simulink model "OpticflowRotation_mod"  (Simulink 7.6)
settings: Solver=ode45  StartTime=0.0  StopTime=inf  FixedStep=1  RelTol=1e-3
undefined symbols (not defined in the file or in its folder): Horn, jet, none, Schunck, videoinput
libraries: dspstat3 x6, simulink x3, dspmtrx3 x2, vipanalysis x2, imaqlib x1, vipsnks x1
settings Model: Creator=pacifist  LastModifiedBy=Administrator
settings SimEventsCC: propDiagAttribOutput=1  propDiagFcnCallOutput=1  propDiagStatOutput=0

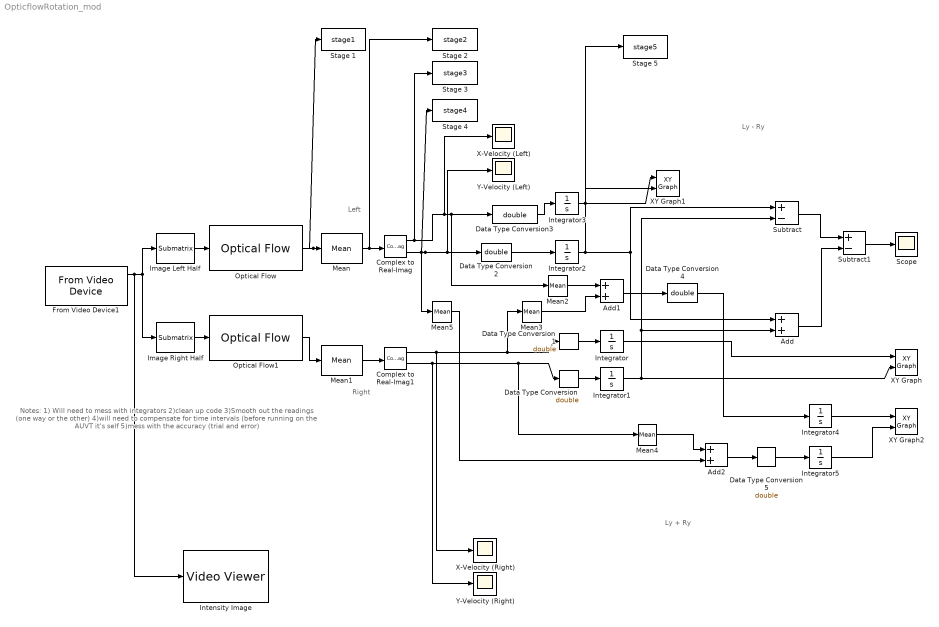
== system OpticflowRotation_mod ==
  note: Notes:
      | 1) Will need to mess with integrators
      | 2)clean up code
      | 3)Smooth out the readings (one way or the other)
      | 4)will need to compensate for time intervals (before running on the AUVT it's self
      | 5)mess with the accuracy (trial and error)
  note: Right
  note: Left
  note: Ly - Ry
  note: Ly + Ry
  Add : Sum
  Add1 : Sum
  Add2 : Sum
  Complex to Real-Imag : ComplexToRealImag
  Complex to Real-Imag1 : ComplexToRealImag
  Data Type Conversion{,1..5} (6 alike) : DataTypeConversion  OutDataTypeStr=double
  From Video Device1 : imaqlib/From Video Device  DialogController=imaqcreatedialog  DialogControllerArgs=DataTag1  DeviceMenu=winvideo 1 (VC0334 USB2.0 Digital Camera)  Device=winvideo 1 (VC0334 USB2.0 Digital Camera)  ObjConstructor=videoinput('winvideo', 1)  VideoFormatMenu=I420_160x120  VideoFormat=I420_160x120  VideoSource=input1  ROIPosition=[0 0 120 160]  EnableHWTrigger=off  TriggerConfiguration=none/none  SampleTime=1/30  OutputPortsMode=Separate color signals  DataType=single  CanDoHWTrigger=no  ReturnedColorSpace=YCbCr  BlockHandle=1940.0005  ROIWidth=160  ROIHeight=120  ROIColumn=0  ROIRow=0  EngXMLPath=C:\Program Files\MATLAB\R2010b\toolbox\imaq\imaq\private  DevXMLPath=C:\Program Files\MATLAB\R2010b\toolbox\imaq\imaqadaptors\win32  EngLibPath=C:\Program Files\MATLAB\R2010b\toolbox\imaq\imaqblks\imaqmex\win32
  Image Left Half : dspmtrx3/Submatrix  RowSpan=All rows  RowStartMode=First  RowStartIndex=1  RowEndMode=Last  RowEndIndex=1  ColSpan=Range of columns  ColStartMode=First  ColStartIndex=1  ColEndMode=Offset from middle  ColEndIndex=-1
  Image Right Half : dspmtrx3/Submatrix  RowSpan=All rows  RowStartMode=First  RowStartIndex=1  RowEndMode=Last  RowEndIndex=1  ColSpan=Range of columns  ColStartMode=Middle  ColStartIndex=1  ColEndMode=Last  ColEndIndex=1
  Integrator{,1..5} (6 alike) : Integrator  LimitOutput=on  UpperSaturationLimit=.01  LowerSaturationLimit=-.01
  Intensity Image : vipsnks/Video Viewer  DialogControllerArgs=DataTag3  inputType=Obsolete7b  imagePorts=One multidimensional signal  useColorMap=off  colormapValue=jet(256)  specRange=off  minInputVal=0  maxInputVal=255  FigPos=[691 710 267 180]  AxisZoom=on  trueSizedOnce=off  OpenAtMdlStart=on
  Mean : dspstat3/Mean  DialogController=dspDDGCreate  DialogControllerArgs=DataTag5  run=off  reset_popup=None  InputProcessing=Columns as channels (frame based)  directionMode=Entire input  dimension=1  treatSBRowAsCol=on  roiEnable=off  roiType=Rectangles  roiPortion=Entire ROI  roiOutput=Individual statistics for each ROI  roiFlag=off  outputDataTypeStr=Inherit: Same as accumulator  outputLastDataTypeStr=Inherit: Same as accumulator  outputMin=[]  outputMax=[]  roundingMode=Floor  overflowMode=off
  Mean1 : dspstat3/Mean  DialogController=dspDDGCreate  DialogControllerArgs=DataTag7  run=off  reset_popup=None  InputProcessing=Columns as channels (frame based)  directionMode=Entire input  dimension=1  treatSBRowAsCol=on  roiEnable=off  roiType=Rectangles  roiPortion=Entire ROI  roiOutput=Individual statistics for each ROI  roiFlag=off  outputDataTypeStr=Inherit: Same as accumulator  outputLastDataTypeStr=Inherit: Same as accumulator  outputMin=[]  outputMax=[]  roundingMode=Floor  overflowMode=off
  Mean2 : dspstat3/Mean  DialogController=dspDDGCreate  DialogControllerArgs=DataTag9  run=off  reset_popup=None  InputProcessing=Columns as channels (frame based)  directionMode=Entire input  dimension=1  treatSBRowAsCol=on  roiEnable=off  roiType=Rectangles  roiPortion=Entire ROI  roiOutput=Individual statistics for each ROI  roiFlag=off  outputDataTypeStr=Inherit: Same as accumulator  outputLastDataTypeStr=Inherit: Same as accumulator  outputMin=[]  outputMax=[]  roundingMode=Floor  overflowMode=off
  Mean3 : dspstat3/Mean  DialogController=dspDDGCreate  DialogControllerArgs=DataTag11  run=off  reset_popup=None  InputProcessing=Columns as channels (frame based)  directionMode=Entire input  dimension=1  treatSBRowAsCol=on  roiEnable=off  roiType=Rectangles  roiPortion=Entire ROI  roiOutput=Individual statistics for each ROI  roiFlag=off  outputDataTypeStr=Inherit: Same as accumulator  outputLastDataTypeStr=Inherit: Same as accumulator  outputMin=[]  outputMax=[]  roundingMode=Floor  overflowMode=off
  Mean4 : dspstat3/Mean  DialogController=dspDDGCreate  DialogControllerArgs=DataTag13  run=off  reset_popup=None  InputProcessing=Columns as channels (frame based)  directionMode=Entire input  dimension=1  treatSBRowAsCol=on  roiEnable=off  roiType=Rectangles  roiPortion=Entire ROI  roiOutput=Individual statistics for each ROI  roiFlag=off  outputDataTypeStr=Inherit: Same as accumulator  outputLastDataTypeStr=Inherit: Same as accumulator  outputMin=[]  outputMax=[]  roundingMode=Floor  overflowMode=off
  Mean5 : dspstat3/Mean  DialogController=dspDDGCreate  DialogControllerArgs=DataTag15  run=off  reset_popup=None  InputProcessing=Columns as channels (frame based)  directionMode=Entire input  dimension=1  treatSBRowAsCol=on  roiEnable=off  roiType=Rectangles  roiPortion=Entire ROI  roiOutput=Individual statistics for each ROI  roiFlag=off  outputDataTypeStr=Inherit: Same as accumulator  outputLastDataTypeStr=Inherit: Same as accumulator  outputMin=[]  outputMax=[]  roundingMode=Floor  overflowMode=off
  Optical Flow : vipanalysis/Optical Flow  DialogController=vipDDGCreate  DialogControllerArgs=DataTag16  SystemSampleTime=-1  method=Horn-Schunck  gradMethod=Difference filter [-1 1]  which2img=Current frame and N-th frame back  N=1  outVelForm=Horizontal and vertical components in complex form  lambda=5  stop_criteria=When maximum number of iterations is reached  maxAllowAbsDiff=eps  maxIter=10  numInports=3  sigmaS=1.5  sigmaW=1  eigTh=0.0039  discardNormalFlow=off  outputCurrentImage=off  prodOutputMode=Binary point scaling  prodOutputWordLength=32  prodOutputFracLength=20  outputMode=Binary point scaling  outputWordLength=32  outputFracLength=20  roundingMode=Nearest  overflowMode=on
      link override Optical Flow Estimation: which2img=Current frame and N-th frame back  outVelForm=Magnitude-squared
  Optical Flow1 : vipanalysis/Optical Flow  DialogController=vipDDGCreate  DialogControllerArgs=DataTag17  SystemSampleTime=-1  method=Horn-Schunck  gradMethod=Difference filter [-1 1]  which2img=Current frame and N-th frame back  N=1  outVelForm=Horizontal and vertical components in complex form  lambda=5  stop_criteria=When maximum number of iterations is reached  maxAllowAbsDiff=eps  maxIter=10  numInports=3  sigmaS=1.5  sigmaW=1  eigTh=0.0039  discardNormalFlow=off  outputCurrentImage=off  prodOutputMode=Binary point scaling  prodOutputWordLength=32  prodOutputFracLength=20  outputMode=Binary point scaling  outputWordLength=32  outputFracLength=20  roundingMode=Nearest  overflowMode=on
      link override Optical Flow Estimation: which2img=Current frame and N-th frame back  outVelForm=Magnitude-squared
  Scope : Scope
      settings: YMin=-0.02  YMax=0.02
  Stage 1 : ToWorkspace  VariableName=stage1  SampleTime=-1  SaveFormat=Array
  Stage 2 : ToWorkspace  VariableName=stage2  SampleTime=-1  SaveFormat=Array
  Stage 3 : ToWorkspace  VariableName=stage3  SampleTime=-1  SaveFormat=Array
  Stage 4 : ToWorkspace  VariableName=stage4  SampleTime=-1  SaveFormat=Array
  Stage 5 : ToWorkspace  VariableName=stage5  SampleTime=-1  SaveFormat=Array
  Subtract : Sum  Inputs=+-
  Subtract1 : Sum  Inputs=+-
  X-Velocity (Left) : Scope
      settings: YMin=-0.02  YMax=0.02
  X-Velocity (Right) : Scope
      settings: YMin=-0.02  YMax=0.02  SaveName=ScopeData3
  XY Graph : simulink/Sinks/XY Graph  SystemSampleTime=-1  xmin=-.01  xmax=.01  ymin=-.01  ymax=.01  st=-1
  XY Graph1 : simulink/Sinks/XY Graph  SystemSampleTime=-1  xmin=-.01  xmax=.01  ymin=-.01  ymax=.01  st=-1
  XY Graph2 : simulink/Sinks/XY Graph  SystemSampleTime=-1  xmin=-.01  xmax=.01  ymin=-.01  ymax=.01  st=-1
  Y-Velocity (Left) : Scope
      settings: YMin=-0.02  YMax=0.02  SaveName=ScopeData2
  Y-Velocity (Right) : Scope
      settings: YMin=-0.02  YMax=0.02  SaveName=ScopeData4
  wires:
  Optical Flow/1 -> Mean/1, Stage 1/1
  Image Left Half/1 -> Optical Flow/1
  From Video Device1/1 -> Image Left Half/1, Image Right Half/1, Intensity Image/1
  Image Right Half/1 -> Optical Flow1/1
  Optical Flow1/1 -> Mean1/1
  Subtract/1 -> Subtract1/1
  Add/1 -> Subtract1/2
  Complex to Real-Imag/2 -> Mean5/1, Stage 4/1, Data Type Conversion2/1, Y-Velocity (Left)/1
  Mean1/1 -> Complex to Real-Imag1/1
  Complex to Real-Imag1/2 -> Data Type Conversion/1, Mean4/1, Y-Velocity (Right)/1
  Subtract1/1 -> Scope/1
  Complex to Real-Imag1/1 -> Data Type Conversion1/1, Mean3/1, X-Velocity (Right)/1
  Complex to Real-Imag/1 -> Stage 3/1, Data Type Conversion3/1, Mean2/1, X-Velocity (Left)/1
  Integrator/1 -> XY Graph/1
  Integrator1/1 -> XY Graph/2, Subtract/2, Add/2
  Mean/1 -> Complex to Real-Imag/1, Stage 2/1
  Integrator2/1 -> Subtract/1, Add/1, XY Graph1/2
  Integrator3/1 -> XY Graph1/1, Stage 5/1
  Data Type Conversion/1 -> Integrator1/1
  Data Type Conversion1/1 -> Integrator/1
  Data Type Conversion2/1 -> Integrator2/1
  Data Type Conversion3/1 -> Integrator3/1
  Mean2/1 -> Add1/1
  Mean3/1 -> Add1/2
  Mean5/1 -> Add2/2
  Mean4/1 -> Add2/1
  Integrator4/1 -> XY Graph2/1
  Integrator5/1 -> XY Graph2/2
  Add1/1 -> Data Type Conversion4/1
  Data Type Conversion4/1 -> Integrator4/1
  Add2/1 -> Data Type Conversion5/1
  Data Type Conversion5/1 -> Integrator5/1
